simulink model "DiagramSimpleSimulink"  (R2019b)
settings: Solver=VariableStepAuto  StartTime=0.0  StopTime=10  MaxStep=0.1  RelTol=1e-3  EnableMultiTasking=on
settings Model: Creator=andre  LastModifiedBy=asmendes
settings DataIOCC: LimitDataPoints=on  SaveFormat=Array  ReturnWorkspaceOutputs=off
settings OptimizationCC: LifeSpan=inf
settings DebuggingCC: UnderspecifiedInitializationDetection=Classic  MergeDetectMultiDrivingBlocksExec=none  SolverPrmCheckMsg=warning  StateNameClashWarn=warning  SFUnexpectedBacktrackingDiag=warning  SFNoUnconditionalDefaultTransitionDiag=warning  SFExecutionAtInitializationDiag=none  ArithmeticOperatorsInVariantConditions=warning
settings HardwareCC: ProdBitPerPointer=32  ProdBitPerSizeT=32  ProdBitPerPtrDiffT=32  ProdLargestAtomicFloat=None  ProdIntDivRoundTo=Undefined  ProdEndianess=Unspecified  ProdWordSize=32  ProdHWDeviceType=32-bit Generic
settings ModelReferenceCC: PropagateSignalLabelsOutOfModel=off
settings SFSimCC: SimUseLocalCustomCode=off  CustomCodeUndefinedFunction=UseInterfaceOnly
settings RTWCC: RTWUseLocalCustomCode=off
settings CodeAppCC: StateflowObjectComments=on
settings GRTTargetCC: TargetLangStandard=C89/C90 (ANSI)  GeneratePreprocessorConditionals=Disable all
settings ConfigComp: CovMetricSettings=dw  CovHtmlReporting=on  CovSaveCumulativeToWorkspaceVar=on  CovSaveSingleToWorkspaceVar=on  CovExternalEMLEnable=off

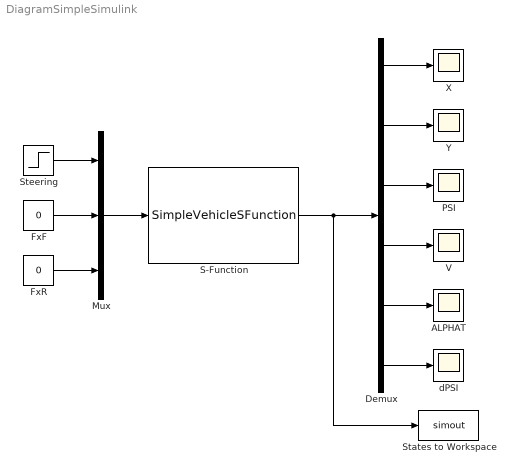
== system DiagramSimpleSimulink ==
  ALPHAT : Scope
  Demux : Demux  Outputs=6
  FxF : Constant  Value=0
  FxR : Constant  Value=0
  Mux : Mux  Inputs=3
  PSI : Scope
  S-Function : S-Function  FunctionName=SimpleVehicleSFunction  SFunctionDeploymentMode=off  EnableBusSupport=off
  States to Workspace : ToWorkspace  VariableName=simout  SaveFormat=Timeseries  SampleTime=-1
  Steering : Step  After=5*pi/180  SampleTime=0
  V : Scope
  X : Scope
  Y : Scope
  dPSI : Scope
  wires:
  FxF/1 -> Mux/2
  FxR/1 -> Mux/3
  Mux/1 -> S-Function/1
  S-Function/1 -> Demux/1, States to Workspace/1
  Demux/1 -> X/1
  Demux/2 -> Y/1
  Demux/3 -> PSI/1
  Demux/4 -> V/1
  Demux/5 -> ALPHAT/1
  Demux/6 -> dPSI/1
  Steering/1 -> Mux/1
